simulink model "Motor_Spindle_with_Load"  (R2023a)
settings: Solver=VariableStepAuto  StartTime=0.0  StopTime=simtime  MaxStep=0.01  RelTol=1e-3
values from neighbouring files (symbols this model uses):
  eta_sp = 0.95    [Model_Values.mat]
  F_L = 5    [Model_Values.mat]
  h_sp = 0.001    [Model_Values.mat]
  i_G = 0.8    [Model_Values.mat]
  J_Mo = 0.005    [Model_Values.mat]
  M = 1    [Model_Values.mat]
  M_Mo = 0.006    [Model_Values.mat]
settings Model: Creator=fycce  LastModifiedBy=fycce
settings DataIOCC: SaveOutput=off  SaveTime=off  ReturnWorkspaceOutputs=off

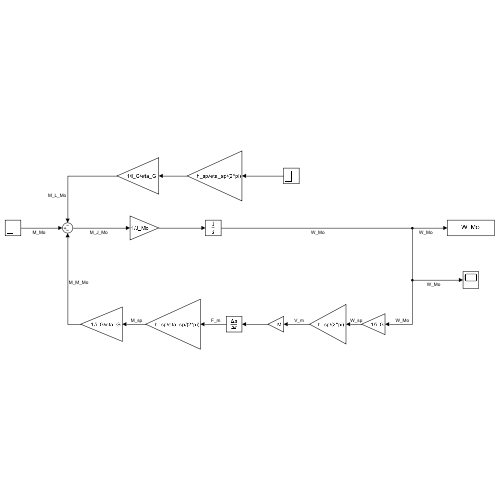
[thumbnail: Simulink's stored preview of the top-level diagram]
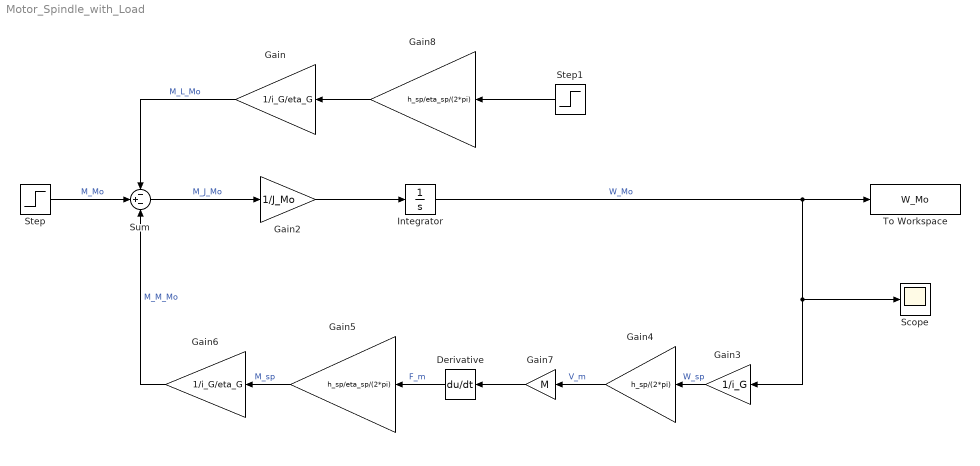
== system Motor_Spindle_with_Load ==
  Derivative : Derivative
  Gain : Gain  Gain=1/i_G/eta_G
  Gain2 : Gain  Gain=1/J_Mo
  Gain3 : Gain  Gain=1/i_G
  Gain4 : Gain  Gain=h_sp/(2*pi)
  Gain5 : Gain  Gain=h_sp/eta_sp/(2*pi)
  Gain6 : Gain  Gain=1/i_G/eta_G
  Gain7 : Gain  Gain=M
  Gain8 : Gain  Gain=h_sp/eta_sp/(2*pi)
  Integrator : Integrator
  Scope : Scope
  Step : Step  After=M_Mo  SampleTime=0
  Step1 : Step  After=F_L  SampleTime=0
  Sum : Sum  Inputs=-+-
  To Workspace : ToWorkspace  VariableName=W_Mo  SaveFormat=Timeseries  SampleTime=-1
  wires:
  Step/1 -> Sum/2  "M_Mo"
  Gain/1 -> Sum/1  "M_L_Mo"
  Gain8/1 -> Gain/1
  Step1/1 -> Gain8/1
  Sum/1 -> Gain2/1  "M_J_Mo"
  Gain2/1 -> Integrator/1
  Integrator/1 -> To Workspace/1, Gain3/1, Scope/1  "W_Mo"
  Gain3/1 -> Gain4/1  "W_sp"
  Derivative/1 -> Gain5/1  "F_m"
  Gain5/1 -> Gain6/1  "M_sp"
  Gain6/1 -> Sum/3  "M_M_Mo"
  Gain4/1 -> Gain7/1  "V_m"
  Gain7/1 -> Derivative/1
